simulink model "assumption"  (R2014b)
settings: Solver=VariableStepDiscrete  StartTime=0.0  StopTime=10.0  RelTol=1e-3
settings Model: Creator=arnaud  LastModifiedBy=hbourbou
settings DataIOCC: SaveFormat=Structure  SignalLoggingSaveFormat=ModelDataLogs
settings OptimizationCC: ExpressionDepthLimit=2147483647
settings DebuggingCC: UnderspecifiedInitializationDetection=Classic  MergeDetectMultiDrivingBlocksExec=none  FcnCallInpInsideContextMsg=EnableAllAsWarning  FrameProcessingCompatibilityMsg=error  StateNameClashWarn=warning
settings GRTTargetCC: CombineOutputUpdateFcns=off  GRTInterface=on

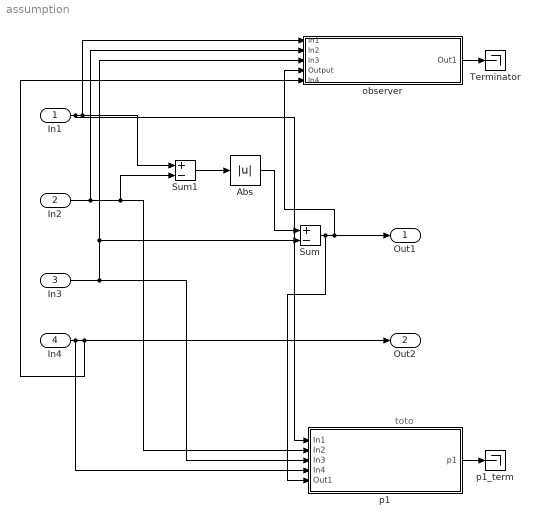
== system assumption ==
  note: toto
  In1 : Inport
  In2 : Inport  Port=2
  In3 : Inport  Port=3
  In4 : Inport  Port=4
  Abs : Abs
  Sum : Sum  Inputs=+-
  Sum1 : Sum  Inputs=+-
  Terminator : Terminator
  observer : Subsystem  TreatAsAtomicUnit=on  mask(Observer){AnnotationType=ensures, ObserverType=ellipsoid}
      mask prompts: AnnotationType "Type of annotation (pre/post...)"; ObserverType "Observer type"
      mask help: Set an observer for the system. The annotation type parameter sets the type of observer: - requires : pre-condition - ensures : post-condition - assert : an assertion - observer : the observer computes a special type of properties
      mask TypeOptions AnnotationType: ensures | requires | assert | observer
      mask Callback AnnotationType:
      | paramStr = get_param(gcb, 'MaskValues');
      | 
      | if strcmp(paramStr{1}(1),'o')
      |     set_param(gcb,'MaskVisibilities',{'on';'on'});
      |     paramStr{2} = 'ellipsoid';
      |     set_param(gcb,'MaskValues',paramStr);
      | else
      |     set_param(gcb,'MaskVisibilities',{'on';'off'});
      | end
      mask Callback ObserverType:
      | paramStr = get_param(gcb, 'MaskValues');
      | 
      | if strcmp(paramStr{1}(1),'observer')
      |     set_param(gcb,'MaskVisibilities',{'on';'on'});
      |     paramStr{2} = 'ellipsoid';
      |     set_param(gcb,'MaskValues',paramStr);
      | else
      |     set_param(gcb,'MaskVisibilities',{'on';'off'});
      | end
      mask Display:
      | color('black')
      | text(0.5, 0.5, ['Property: ''' get_param(gcb,'name') ''''], 'horizontalAlignment', 'center');
      | text(0.99, 0.03, '{\bf\fontsize{12}CEX}', 'hor', 'right', 'ver', 'bottom', 'texmode', 'on');
  p1 : Subsystem  TreatAsAtomicUnit=on  mask(Observer){AnnotationType=ensures, ObserverType=[]}
      mask prompts: AnnotationType "Type of annotation (pre/post...)"; ObserverType "Observer type"
      mask help:
      | Set an observer for the system.
      | The annotation type parameter sets the type of observer:
      | - requires : pre-condition
      | - ensures : post-condition
      | - assert : an assertion
      | - observer : the observer computes a special type of properties
      mask TypeOptions AnnotationType: ensures | requires | assert | observer
      mask Callback AnnotationType:
      | paramStr = get_param(gcb, 'MaskValues');
      | if strcmp(paramStr{1}(1),'o')
      | set_param(gcb,'MaskVisibilities',{'on';'on'});
      | paramStr{2} = 'ellipsoid';
      | set_param(gcb,'MaskValues',paramStr);
      | else
      | set_param(gcb,'MaskVisibilities',{'on';'off'});
      | end
      | clear paramStr;
      mask Callback ObserverType:
      | paramStr = get_param(gcb, 'MaskValues');
      | if strcmp(paramStr{1}(1),'o')
      | set_param(gcb,'MaskVisibilities',{'on';'on'});
      | paramStr{2} = 'ellipsoid';
      | set_param(gcb,'MaskValues',paramStr);
      | else
      | set_param(gcb,'MaskVisibilities',{'on';'off'});
      | end
      | clear paramStr;
      mask Display:
      | color('red')
      | text(0.5, 0.5, ['CoCoSpec: ''' get_param(gcb,'name') ''''], 'horizontalAlignment', 'center');
      | text(0.99, 0.03, '{\bf\fontsize{12}TO BE VERIFIED}', 'hor', 'right', 'ver', 'bottom', 'texmode', 'on');
  p1_term : Terminator
  Out1 : Outport
  Out2 : Outport  Port=2
  wires:
  observer/1(Out1) -> Terminator/1
  In2/1 -> p1/2(In2), Sum1/2, observer/2(In2)
  In1/1 -> Sum1/1, observer/1(In1), p1/1(In1)
  Sum/1 -> Out1/1, observer/4(Output), p1/5(Out1)
  Sum1/1 -> Abs/1
  Abs/1 -> Sum/1
  In3/1 -> Sum/2, observer/3(In3), p1/3(In3)
  In4/1 -> Out2/1, observer/5(In4), p1/4(In4)
  p1/1(p1) -> p1_term/1

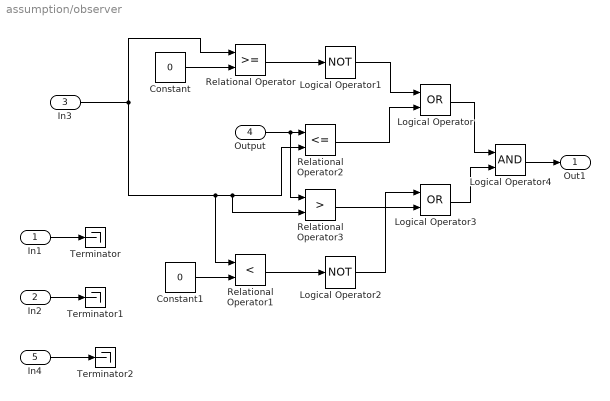
== system assumption/observer ==
  In1 : Inport
  In2 : Inport  Port=2
  In3 : Inport  Port=3
      settings: AttributesFormatString=assume In3 > 0.0;
  Output : Inport  Port=4
  In4 : Inport  Port=5
  Constant : Constant  Value=0
  Constant1 : Constant  Value=0
  Logical Operator : Logic  Operator=OR  AllPortsSameDT=off  OutDataTypeStr=boolean
  Logical Operator1 : Logic  Operator=NOT  AllPortsSameDT=off  OutDataTypeStr=boolean
  Logical Operator2 : Logic  Operator=NOT  AllPortsSameDT=off  OutDataTypeStr=boolean
  Logical Operator3 : Logic  Operator=OR  AllPortsSameDT=off  OutDataTypeStr=boolean
  Logical Operator4 : Logic  AllPortsSameDT=off  OutDataTypeStr=boolean
  Relational Operator : RelationalOperator  OutDataTypeStr=boolean
  Relational Operator1 : RelationalOperator  Operator=<  OutDataTypeStr=boolean
  Relational Operator2 : RelationalOperator  Operator=<=  OutDataTypeStr=boolean
  Relational Operator3 : RelationalOperator  Operator=>  OutDataTypeStr=boolean
  Terminator : Terminator
  Terminator1 : Terminator
  Terminator2 : Terminator
  Out1 : Outport
  wires:
  In3/1 -> Relational Operator3/2, Relational Operator2/2, Relational Operator1/1, Relational Operator/1
  Constant/1 -> Relational Operator/2
  Constant1/1 -> Relational Operator1/2
  Relational Operator/1 -> Logical Operator1/1
  Relational Operator1/1 -> Logical Operator2/1
  Logical Operator2/1 -> Logical Operator3/1
  Logical Operator1/1 -> Logical Operator/1
  Output/1 -> Relational Operator3/1, Relational Operator2/1
  Relational Operator2/1 -> Logical Operator/2
  Relational Operator3/1 -> Logical Operator3/2
  Logical Operator3/1 -> Logical Operator4/2
  Logical Operator/1 -> Logical Operator4/1
  Logical Operator4/1 -> Out1/1
  In2/1 -> Terminator1/1
  In1/1 -> Terminator/1
  In4/1 -> Terminator2/1

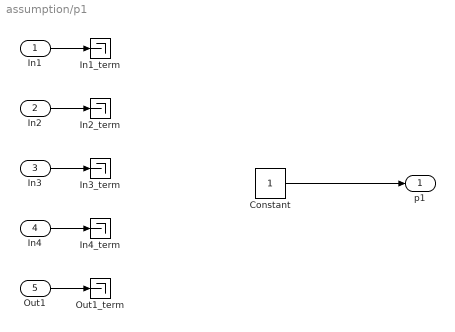
== system assumption/p1 ==
  In1 : Inport
  In2 : Inport  Port=2
  In3 : Inport  Port=3
  In4 : Inport  Port=4
  Out1 : Inport  Port=5
  Constant : Constant  OutDataTypeStr=boolean
  In1_term : Terminator
  In2_term : Terminator
  In3_term : Terminator
  In4_term : Terminator
  Out1_term : Terminator
  p1 : Outport
  wires:
  In1/1 -> In1_term/1
  In2/1 -> In2_term/1
  In3/1 -> In3_term/1
  In4/1 -> In4_term/1
  Out1/1 -> Out1_term/1
  Constant/1 -> p1/1
